simulink model "LKASampleSimulink"  (Simulink 9.1)
settings: Solver=ode1  StartTime=0.0  StopTime=inf  FixedStep=0.001  RelTol=1e-3
model workspace (MAT data in the model file):
  ParaDataStoreNum = Simulink.Parameter
  ParaDataStoreNum.DataType = 'int32'
  ParaDataStoreNum.Complexity = 'real'
  ParaDataStoreNum.Dimensions = [0 0]
InitFcn:
  | load('LKAExampleVariable.mat')
values from neighbouring files (symbols this model uses):
  DataStoreNumPara = 0    [LKAExampleVariable.mat]
  headwayOffset = 3.7    [LKAExampleVariable.mat]
undefined symbols (not defined in the file or in its folder): azimuth_angle, BrStatus, elevation_angle, GroundTruth_Objects, heading, id, Lane_Car_Distance_Left, Lane_Car_Distance_Right, Lane_Class, Lane_Coefficient_C0, Lane_Coefficient_C1, Lane_Coefficient_C2, Lane_Coefficient_C3, Lane_Curvature, Lane_Distance, Lane_ID, LaneInfoPerception, range_bbox, range_center, shape, time, Timestamp, type, velocity, width
libraries: mpcadaslib x1
(part 1 of 2)
Description:
  | 22222
settings Model: Creator=15751  LastModifiedBy=jwd  EnablePacing=on
settings DataIOCC: SaveFormat=Dataset  ReturnWorkspaceOutputs=on
settings DebuggingCC: UnderspecifiedInitializationDetection=Simplified  MergeDetectMultiDrivingBlocksExec=error  MultiTaskRateTransMsg=warning  SFUnexpectedBacktrackingDiag=error  SFNoUnconditionalDefaultTransitionDiag=error
settings HardwareCC: ProdBitPerPointer=64  ProdBitPerSizeT=64  ProdBitPerPtrDiffT=64  ProdLargestAtomicFloat=Float  ProdIntDivRoundTo=Zero  ProdEndianess=LittleEndian  ProdWordSize=64  ProdHWDeviceType=Intel->x86-64 (Windows64)
settings ModelReferenceCC: PropagateSignalLabelsOutOfModel=on
settings SFSimCC: SimUseLocalCustomCode=on
settings RTWCC: RTWUseLocalCustomCode=on
settings GRTTargetCC: TargetLangStandard=C99 (ISO)  CombineOutputUpdateFcns=on  GRTInterface=off
settings ConfigComp: CovMetricSettings=dwe  CovSaveCumulativeToWorkspaceVar=off  CovSaveSingleToWorkspaceVar=off  CovExternalEMLEnable=on

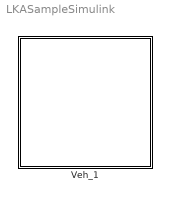
== system LKASampleSimulink ==
  Veh_1 : Subsystem  Tag=PanoSim_System
      mask Display: image(imread('Sedan_2.jpg'));color('white');text(0,0,'Veh_1','HorizontalAlignment','left','verticalAlignment','bottom');color('red');text(0.1,0.1,'P','HorizontalAlignment','right','verticalAlignment','top');

== system LKASampleSimulink/Veh_1 ==
  Algorithm : Subsystem
  AlgorithmControl : Subsystem
  ComplexVehicleModel : Subsystem
  Data Store Memory1 : DataStoreMemory  DataStoreName=DataStore_EGO_ALL  ReadBeforeWriteMsg=warning  WriteAfterWriteMsg=warning  WriteAfterReadMsg=warning  InitialValue=zeros(295,1)  ShowAdditionalParam=off  Dimensions=295
      settings: LockScale=on
  Data Store Memory2 : DataStoreMemory  DataStoreName=DataStore_COCKPIT_CONTROL  ReadBeforeWriteMsg=warning  WriteAfterWriteMsg=warning  WriteAfterReadMsg=warning  InitialValue=[0,0,0,0,0,0]  ShowAdditionalParam=off  Dimensions=6
      settings: LockScale=on
  Data Store Memory : DataStoreMemory  DataStoreName=DataStore_Ego_Control  ReadBeforeWriteMsg=warning  WriteAfterWriteMsg=warning  WriteAfterReadMsg=warning  InitialValue=[0,0,0,0,0,0]  ShowAdditionalParam=off  Dimensions=6
      settings: LockScale=on
  DriverModel : Subsystem  Tag=PanoSim_System
      mask Display: image(imread('driver.jpg'))
  GlobalVariable : Subsystem
  Sensors : Subsystem
  VehicleDataBus : Subsystem
  wires:
  Algorithm/3(LogDataOutput) -> VehicleDataBus/4(LogDataInput)
  Algorithm/2(GlobalVariableOutput) -> VehicleDataBus/2(GlobalVariable)
  Algorithm/1(ControlOutput) -> ComplexVehicleModel/1(Control)
  AlgorithmControl/1(AlgorithmControlOut) -> Algorithm/5(AlgorithmControlInput)
  GlobalVariable/1(Value) -> Algorithm/4(GlobalVariableInput)
  Sensors/1(SensorsOut) -> Algorithm/3(SensorsInput)
  DriverModel/1(DriverOut) -> Algorithm/2(ControlInput)
  [VehicleDynOut] -> Algorithm/1(VehDynInput)
  ComplexVehicleModel/1(Vehicle_Out) -> [VehicleDynOut], VehicleDataBus/1(VehicleDynOut)
  GlobalVariable/2(Original) -> VehicleDataBus/3(GlobalVariableOriginal)
  [VehicleDynOut] -> DriverModel/1(In1)

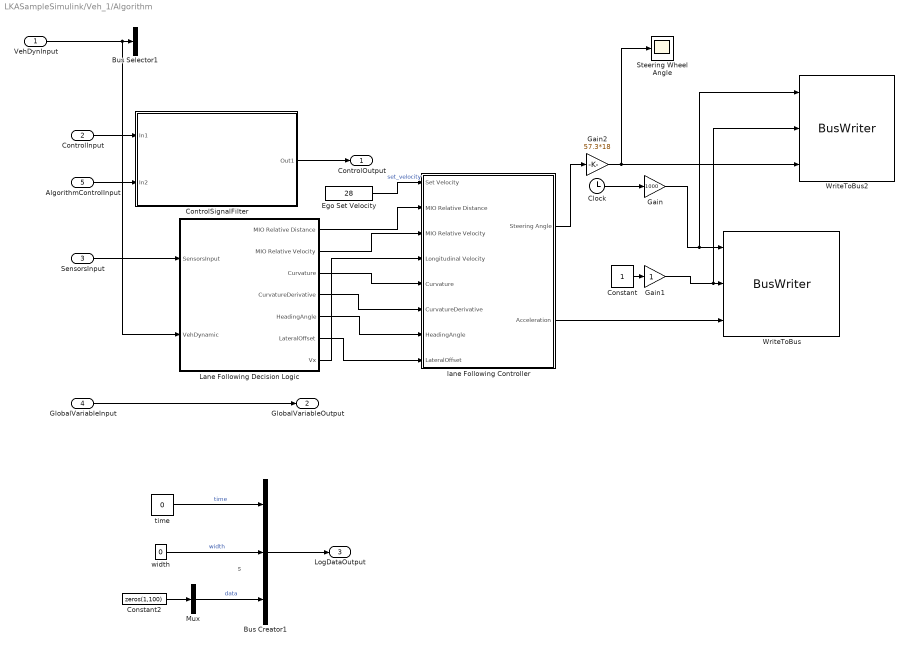
== system LKASampleSimulink/Veh_1/Algorithm ==
  note: s
  VehDynInput : Inport
  ControlInput : Inport  Port=2
  SensorsInput : Inport  Port=3
  GlobalVariableInput : Inport  Port=4
  AlgorithmControlInput : Inport  Port=5
  Bus Creator1 : BusCreator  Inputs=3
  Bus Selector1 : BusSelector  OutputSignals=ego
  Clock : Clock
  Constant : Constant
  Constant2 : Constant  Value=zeros(1,100)
  ControlSignalFilter : Subsystem
  Ego Set Velocity : Constant  Value=28  SampleTime=0.1
  Gain : Gain  Gain=1000  OutDataTypeStr=int32
  Gain1 : Gain  OutDataTypeStr=uint8
  Gain2 : Gain  Gain=57.3*18  OutDataTypeStr=double
  Lane Following Decision Logic : Subsystem
  Mux : Mux  Inputs=[100,]
  Steering Wheel Angle : Scope
  WriteToBus : S-Function  FunctionName=BusWriter  Parameters='xDriver_accel_input','time@i,valid@b,accel@d','0.01','0.0'  SFunctionDeploymentMode=off  EnableBusSupport=off
  WriteToBus2 : S-Function  FunctionName=BusWriter  Parameters='ego_control.steer','time@i,valid@b,steer@d','0.01','0.0'  SFunctionDeploymentMode=off  EnableBusSupport=off
  lane Following Controller : Subsystem
  time : Constant  Value=0
  width : Constant  Value=0
  ControlOutput : Outport  VectorParamsAs1DForOutWhenUnconnected=off
  GlobalVariableOutput : Outport  Port=2  VectorParamsAs1DForOutWhenUnconnected=off
  LogDataOutput : Outport  Port=3  VectorParamsAs1DForOutWhenUnconnected=off
  wires:
  VehDynInput/1 -> Lane Following Decision Logic/2(VehDynamic), Bus Selector1/1
  ControlInput/1 -> ControlSignalFilter/1(In1)
  ControlSignalFilter/1(Out1) -> ControlOutput/1
  GlobalVariableInput/1 -> GlobalVariableOutput/1
  time/1 -> Bus Creator1/1  "time"
  Bus Creator1/1 -> LogDataOutput/1
  Constant2/1 -> Mux/1
  Mux/1 -> Bus Creator1/3  "data"
  width/1 -> Bus Creator1/2  "width"
  AlgorithmControlInput/1 -> ControlSignalFilter/2(In2)
  Ego Set Velocity/1 -> lane Following Controller/1(Set Velocity)  "set_velocity"
  Lane Following Decision Logic/1(MIO Relative Distance) -> lane Following Controller/2(MIO Relative Distance)
  Lane Following Decision Logic/2(MIO Relative Velocity) -> lane Following Controller/3(MIO Relative Velocity)
  Lane Following Decision Logic/3(Curvature) -> lane Following Controller/5(Curvature)
  Lane Following Decision Logic/6(LateralOffset) -> lane Following Controller/8(LateralOffset)
  SensorsInput/1 -> Lane Following Decision Logic/1(SensorsInput)
  lane Following Controller/1(Steering Angle) -> Gain2/1
  lane Following Controller/2(Acceleration) -> WriteToBus/3
  Gain/1 -> WriteToBus2/1, WriteToBus/1
  Clock/1 -> Gain/1
  Gain1/1 -> WriteToBus2/2, WriteToBus/2
  Constant/1 -> Gain1/1
  Lane Following Decision Logic/7(Vx) -> lane Following Controller/4(Longitudinal Velocity)
  Lane Following Decision Logic/5(HeadingAngle) -> lane Following Controller/7(HeadingAngle)
  Lane Following Decision Logic/4(CurvatureDerivative) -> lane Following Controller/6(CurvatureDerivative)
  Gain2/1 -> Steering Wheel Angle/1, WriteToBus2/3

== system LKASampleSimulink/Veh_1/AlgorithmControl ==
  Bus{,2..5} (5 alike) : BusCreator  Inputs=3
  Bus1 : BusCreator  Inputs=5
  brake : S-Function  FunctionName=BusReader  Parameters='ego_control.brake','time@i,valid@b,brake@d','0.001','0.0'  SFunctionDeploymentMode=off  EnableBusSupport=off
  gear : S-Function  FunctionName=BusReader  Parameters='ego_control.gear','time@i,valid@b,gear@i','0.001','0.0'  SFunctionDeploymentMode=off  EnableBusSupport=off
  mode : S-Function  FunctionName=BusReader  Parameters='ego_control.mode','time@i,valid@b,mode@i','0.001','0.0'  SFunctionDeploymentMode=off  EnableBusSupport=off
  steer : S-Function  FunctionName=BusReader  Parameters='ego_control.steer','time@i,valid@b,steer@d','0.001','0.0'  SFunctionDeploymentMode=off  EnableBusSupport=off
  throttle : S-Function  FunctionName=BusReader  Parameters='ego_control.throttle','time@i,valid@b,throttle@d','0.001','0.0'  SFunctionDeploymentMode=off  EnableBusSupport=off
  AlgorithmControlOut : Outport  VectorParamsAs1DForOutWhenUnconnected=off
  wires:
  Bus1/1 -> AlgorithmControlOut/1
  Bus5/1 -> Bus1/1  "throttle"
  Bus4/1 -> Bus1/5  "gear"
  Bus3/1 -> Bus1/4  "mode"
  Bus2/1 -> Bus1/3  "steer"
  Bus/1 -> Bus1/2  "brake"
  gear/3 -> Bus4/3  "value"
  gear/2 -> Bus4/2  "valid"
  gear/1 -> Bus4/1  "time"
  mode/3 -> Bus3/3  "value"
  mode/2 -> Bus3/2  "valid"
  mode/1 -> Bus3/1  "time"
  steer/1 -> Bus2/1  "time"
  brake/1 -> Bus/1  "time"
  throttle/1 -> Bus5/1  "time"
  throttle/3 -> Bus5/3  "value"
  brake/3 -> Bus/3  "value"
  steer/3 -> Bus2/3  "value"
  throttle/2 -> Bus5/2  "valid"
  brake/2 -> Bus/2  "valid"
  steer/2 -> Bus2/2  "valid"

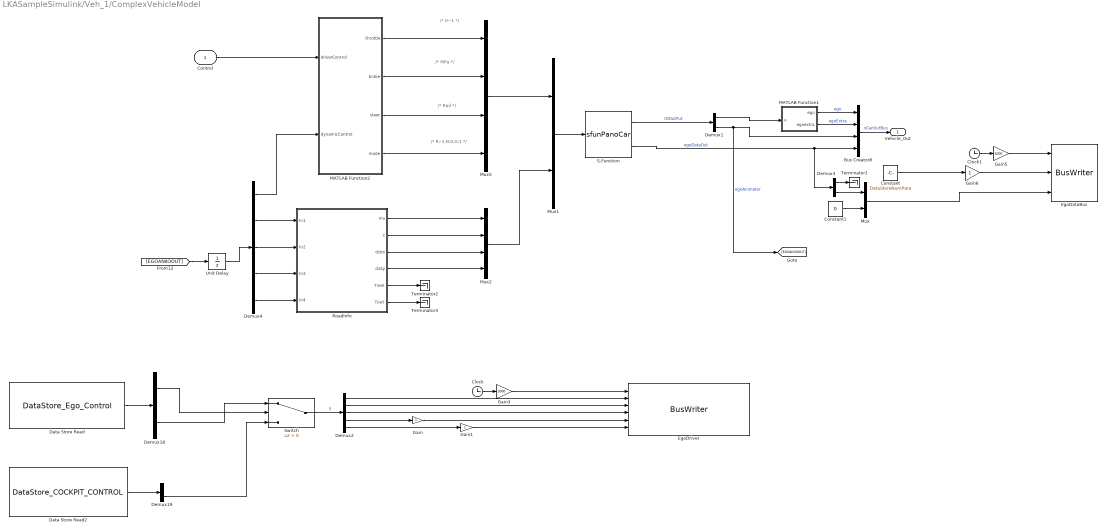
== system LKASampleSimulink/Veh_1/ComplexVehicleModel ==
  note: /* MPa */
  note: /* 0~1 */
  note: /* R:-1,N:0,D:1 */
  note: /* Rad */
  Control : Inport
  Bus Creator8 : BusCreator  Inputs=4
  Clock : Clock
  Clock1 : Clock
  Constant : Constant  Value=DataStoreNumPara  VectorParams1D=off  OutDataTypeStr=double
  Constant1 : Constant  Value=0
  Data Store Read : DataStoreRead  DataStoreName=DataStore_Ego_Control
  Data Store Read2 : DataStoreRead  DataStoreName=DataStore_COCKPIT_CONTROL
  Demux1 : Demux  Outputs=[19,57]
  Demux18 : Demux  Outputs=[1,5]
  Demux19 : Demux  Outputs=[1,5]
  Demux2 : Demux  Outputs=5
  Demux3 : Demux  Outputs=[1,499]
  Demux4 : Demux  Outputs=[5,13,13,13,13]
  EgoDataBus : S-Function  FunctionName=BusWriter  Parameters='ego_data','time@i,500@[,data@d','0.01','0.0'  SFunctionDeploymentMode=off  EnableBusSupport=off
  EgoDriver : S-Function  FunctionName=BusWriter  Parameters='ego_driver','time@i,throttle@d,brake@d,steer@d,mode@i,gear@i','0.01','0.0'  SFunctionDeploymentMode=off  EnableBusSupport=off
  Gain : Gain  OutDataTypeStr=int32
  Gain1 : Gain  OutDataTypeStr=int32
  Gain3 : Gain  Gain=1000  OutDataTypeStr=Inherit: Inherit via back propagation  RndMeth=Nearest
  Gain5 : Gain  Gain=1000  OutDataTypeStr=Inherit: Inherit via back propagation  RndMeth=Nearest
  Gain6 : Gain  OutDataTypeStr=int32
  MATLAB Function1 : MATLAB Function  TreatAsAtomicUnit=on
  MATLAB Function2 : MATLAB Function  TreatAsAtomicUnit=on
  Mux : Mux  Inputs=[499,1]
  Mux1 : Mux  Inputs=[4,16]
  Mux2 : Mux
  Mux5 : Mux
  RoadInfo : Subsystem
  S-Function : S-Function  FunctionName=sfunPanoCar  SFunctionDeploymentMode=off  EnableBusSupport=off
  Switch : Switch  Criteria=u2 > Threshold
  Terminator1 : Terminator
  Terminator2 : Terminator
  Terminator3 : Terminator
  Unit Delay : UnitDelay  SampleTime=-1  HasFrameUpgradeWarning=on
  Vehicle_Out : Outport
  wires:
  Demux19/2 -> Switch/3
  Demux18/2 -> Switch/1
  Demux18/1 -> Switch/2
  MATLAB Function2/4(mode) -> Mux5/4
  MATLAB Function2/3(steer) -> Mux5/3
  MATLAB Function2/2(brake) -> Mux5/2
  MATLAB Function2/1(throttle) -> Mux5/1
  Demux4/4 -> RoadInfo/3(In3)
  Demux4/1 -> MATLAB Function2/2(dynamicControl)
  Demux4/2 -> RoadInfo/1(In1)
  Demux4/5 -> RoadInfo/4(In4)
  Unit Delay/1 -> Demux4/1
  Demux4/3 -> RoadInfo/2(In2)
  Mux/1 -> EgoDataBus/3
  Constant1/1 -> Mux/2
  Demux3/2 -> Mux/1
  Demux3/1 -> Terminator1/1
  Constant/1 -> Gain6/1
  Gain5/1 -> EgoDataBus/1
  Clock1/1 -> Gain5/1
  Gain6/1 -> EgoDataBus/2
  Data Store Read2/1 -> Demux19/1
  Data Store Read/1 -> Demux18/1
  Switch/1 -> Demux2/1  "5"
  Demux1/2 -> Bus Creator8/3, [EGOANIIOOUT]  "egoAnimator"
  MATLAB Function1/1(ego) -> Bus Creator8/1  "ego"
  Demux1/1 -> MATLAB Function1/1(u)
  MATLAB Function1/2(egoextra) -> Bus Creator8/2  "egoExtra"
  RoadInfo/6(TireY) -> Terminator3/1
  RoadInfo/5(TireX) -> Terminator2/1
  S-Function/2 -> Bus Creator8/4, Demux3/1  "egoDataOut"
  Gain1/1 -> EgoDriver/6
  Gain/1 -> EgoDriver/5
  Demux2/4 -> Gain/1
  Demux2/2 -> EgoDriver/3
  Control/1 -> MATLAB Function2/1(driverControl)
  Demux2/1 -> EgoDriver/2
  Demux2/3 -> EgoDriver/4
  Demux2/5 -> Gain1/1
  Gain3/1 -> EgoDriver/1
  Mux1/1 -> S-Function/1
  S-Function/1 -> Demux1/1  "IOOutPut"
  Bus Creator8/1 -> Vehicle_Out/1  "xCarOutBus"
  Mux5/1 -> Mux1/1
  Clock/1 -> Gain3/1
  Mux2/1 -> Mux1/2
  RoadInfo/3(dzdx) -> Mux2/3
  RoadInfo/1(mu) -> Mux2/1
  RoadInfo/2(z) -> Mux2/2
  RoadInfo/4(dzdy) -> Mux2/4
  [EGOANIIOOUT] -> Unit Delay/1

== system LKASampleSimulink/Veh_1/DriverModel ==
  In1 : Inport
  DriverFilter : Subsystem
  DriverOut : Outport  VectorParamsAs1DForOutWhenUnconnected=off
  wires:
  DriverFilter/1(DriverOut) -> DriverOut/1

== system LKASampleSimulink/Veh_1/GlobalVariable ==
  Bus : BusCreator  Inputs=2
  Variable : Subsystem
  Value : Outport  VectorParamsAs1DForOutWhenUnconnected=off
  Original : Outport  Port=2  VectorParamsAs1DForOutWhenUnconnected=off
  wires:
  Bus/1 -> Original/1
  Variable/2(Out2) -> Bus/2  "Time"
  Variable/1(Out1) -> Value/1, Bus/1  "Value"

== system LKASampleSimulink/Veh_1/Sensors ==
  GroundTruth_Objects.0 : Subsystem
  LaneInfoPerception.0 : Subsystem
  SensorsBusCreator : BusCreator  Inputs=LaneInfoPerception.0,GroundTruth_Objects.0
  sensor_template : Subsystem  Commented=on
  SensorsOut : Outport  VectorParamsAs1DForOutWhenUnconnected=off
  wires:
  SensorsBusCreator/1 -> SensorsOut/1
  GroundTruth_Objects.0/1(SensorOut) -> SensorsBusCreator/2  "GroundTruth_Objects.0"
  LaneInfoPerception.0/1(SensorOut) -> SensorsBusCreator/1  "LaneInfoPerception.0"

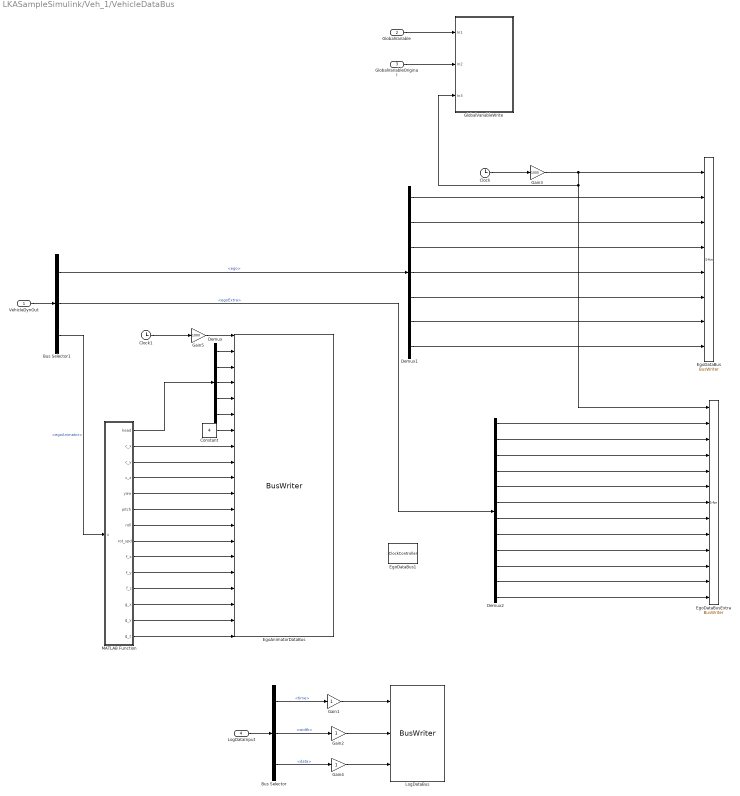
== system LKASampleSimulink/Veh_1/VehicleDataBus ==
  VehicleDynOut : Inport
  GlobalVariable : Inport  Port=2
  GlobalVariableOriginal : Inport  Port=3
  LogDataInput : Inport  Port=4
  Bus Selector : BusSelector  OutputSignals=time,width,data
  Bus Selector1 : BusSelector  OutputSignals=ego,egoExtra,egoAnimator
  Clock : Clock
  Clock1 : Clock
  Constant : Constant  Value=4  OutDataTypeStr=int32
  Demux : Demux  Outputs=5
  Demux1 : Demux  Outputs=7
  Demux2 : Demux  Outputs=12
  EgoAnimatorDataBus : S-Function  FunctionName=BusWriter  Parameters='ego_animator','time@i,rot_spd@d,trans_gear@d,throttle@d,master@d,str@d,4@[,center_x@d,center_y@d,center_z@d,yaw@d,pitch@d,roll@d,rotation_spd@d,force_tire_x@d,force_tire_y@d,force_tire_z@d,gnd_x@d,gnd_y@d,gnd_z@d','0.01','0.0'  SFunctionDeploymentMode=off  EnableBusSupport=off
  EgoDataBus : S-Function  FunctionName=BusWriter  Parameters='ego','time@i,x@d,y@d,z@d,yaw@d,pitch@d,roll@d,speed@d','0.01','0.0'  SFunctionDeploymentMode=off  EnableBusSupport=off
  EgoDataBus1 : S-Function  FunctionName=ClockController  Parameters='step','0.01','0.0'  SFunctionDeploymentMode=off  EnableBusSupport=off
  EgoDataBusExtra : S-Function  FunctionName=BusWriter  Parameters='ego_extra','time@i,VX@d,VY@d,VZ@d,AVx@d,AVy@d,AVz@d,Ax@d,Ay@d,Az@d,AAx@d,AAy@d,AAz@d','0.01','0.0'  SFunctionDeploymentMode=off  EnableBusSupport=off
  Gain1 : Gain  OutDataTypeStr=int32  RndMeth=Nearest
  Gain2 : Gain  OutDataTypeStr=int32  RndMeth=Nearest
  Gain3 : Gain  Gain=1000  OutDataTypeStr=Inherit: Inherit via back propagation  RndMeth=Nearest
  Gain4 : Gain  OutDataTypeStr=double  RndMeth=Nearest
  Gain5 : Gain  Gain=1000  OutDataTypeStr=Inherit: Inherit via back propagation  RndMeth=Nearest
  GlobalVariableWrite : Subsystem
  LogDataBus : S-Function  FunctionName=BusWriter  Parameters='data','time@i,100@[,data@d','0.01','0.0'  SFunctionDeploymentMode=off  EnableBusSupport=off
  MATLAB Function : MATLAB Function  TreatAsAtomicUnit=on
  wires:
  Demux/5 -> EgoAnimatorDataBus/6
  MATLAB Function/14(g_z) -> EgoAnimatorDataBus/20
  MATLAB Function/13(g_y) -> EgoAnimatorDataBus/19
  MATLAB Function/12(g_x) -> EgoAnimatorDataBus/18
  MATLAB Function/11(f_z) -> EgoAnimatorDataBus/17
  MATLAB Function/10(f_y) -> EgoAnimatorDataBus/16
  MATLAB Function/9(f_x) -> EgoAnimatorDataBus/15
  MATLAB Function/8(rot_spd) -> EgoAnimatorDataBus/14
  MATLAB Function/7(roll) -> EgoAnimatorDataBus/13
  MATLAB Function/6(pitch) -> EgoAnimatorDataBus/12
  MATLAB Function/5(yaw) -> EgoAnimatorDataBus/11
  MATLAB Function/4(c_z) -> EgoAnimatorDataBus/10
  MATLAB Function/3(c_y) -> EgoAnimatorDataBus/9
  MATLAB Function/2(c_x) -> EgoAnimatorDataBus/8
  Constant/1 -> EgoAnimatorDataBus/7
  Demux/4 -> EgoAnimatorDataBus/5
  Demux/3 -> EgoAnimatorDataBus/4
  Demux/2 -> EgoAnimatorDataBus/3
  Demux/1 -> EgoAnimatorDataBus/2
  MATLAB Function/1(head) -> Demux/1
  Gain5/1 -> EgoAnimatorDataBus/1
  Clock1/1 -> Gain5/1
  Bus Selector1/3 -> MATLAB Function/1(u)  "<egoAnimator>"
  Bus Selector1/2 -> Demux2/1  "<egoExtra>"
  Bus Selector1/1 -> Demux1/1  "<ego>"
  Gain2/1 -> LogDataBus/2
  Bus Selector/2 -> Gain2/1  "<width>"
  Gain4/1 -> LogDataBus/3
  Bus Selector/1 -> Gain1/1  "<time>"
  Bus Selector/3 -> Gain4/1  "<data>"
  Gain1/1 -> LogDataBus/1
  LogDataInput/1 -> Bus Selector/1
  GlobalVariableOriginal/1 -> GlobalVariableWrite/2(In2)
  Gain3/1 -> EgoDataBus/1, EgoDataBusExtra/1, GlobalVariableWrite/3(In3)
  GlobalVariable/1 -> GlobalVariableWrite/1(In1)
  Demux2/12 -> EgoDataBusExtra/13
  Demux2/11 -> EgoDataBusExtra/12
  Demux2/10 -> EgoDataBusExtra/11
  Demux2/9 -> EgoDataBusExtra/10
  Demux2/8 -> EgoDataBusExtra/9
  Demux2/7 -> EgoDataBusExtra/8
  Demux2/6 -> EgoDataBusExtra/7
  Demux2/5 -> EgoDataBusExtra/6
  Demux2/4 -> EgoDataBusExtra/5
  Demux2/3 -> EgoDataBusExtra/4
  Demux2/2 -> EgoDataBusExtra/3
  Demux2/1 -> EgoDataBusExtra/2
  VehicleDynOut/1 -> Bus Selector1/1
  Clock/1 -> Gain3/1
  Demux1/1 -> EgoDataBus/2
  Demux1/2 -> EgoDataBus/3
  Demux1/3 -> EgoDataBus/4
  Demux1/4 -> EgoDataBus/5
  Demux1/5 -> EgoDataBus/6
  Demux1/6 -> EgoDataBus/7
  Demux1/7 -> EgoDataBus/8

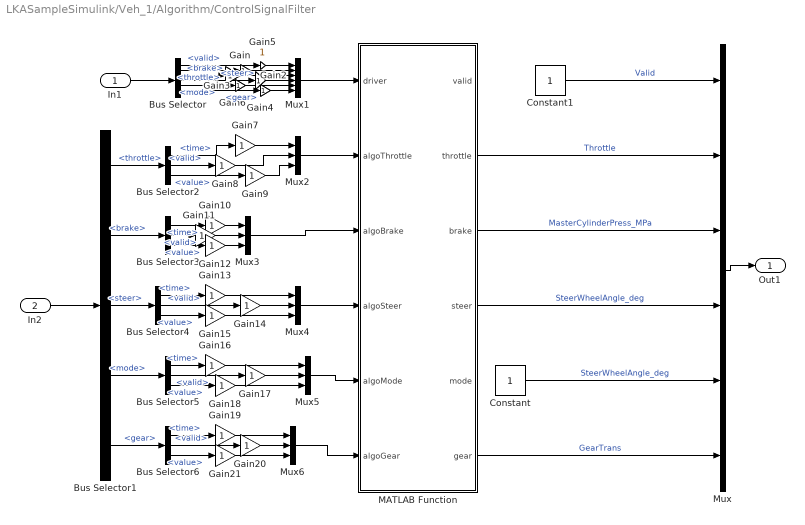
== system LKASampleSimulink/Veh_1/Algorithm/ControlSignalFilter ==
  In1 : Inport
  In2 : Inport  Port=2
  Bus Selector : BusSelector  OutputSignals=valid,throttle,brake,steer,mode,gear
  Bus Selector1 : BusSelector  OutputSignals=throttle,brake,steer,mode,gear
  Bus Selector{2..6} (5 alike) : BusSelector  OutputSignals=time,valid,value
  Constant : Constant
  Constant1 : Constant
  Gain{,2..21} (21 alike) : Gain  OutDataTypeStr=double
  MATLAB Function : MATLAB Function  TreatAsAtomicUnit=on
  Mux : Mux  Inputs=6
  Mux1 : Mux  Inputs=6
  Mux{2..6} (5 alike) : Mux  Inputs=3
  Out1 : Outport  VectorParamsAs1DForOutWhenUnconnected=off
  wires:
  In1/1 -> Bus Selector/1
  Mux/1 -> Out1/1
  MATLAB Function/2(throttle) -> Mux/2  "Throttle"
  MATLAB Function/4(steer) -> Mux/4  "SteerWheelAngle_deg"
  Constant1/1 -> Mux/1  "Valid"
  MATLAB Function/6(gear) -> Mux/6  "GearTrans"
  In2/1 -> Bus Selector1/1
  Bus Selector1/1 -> Bus Selector2/1  "<throttle>"
  Bus Selector1/2 -> Bus Selector3/1  "<brake>"
  Bus Selector1/3 -> Bus Selector4/1  "<steer>"
  Bus Selector1/4 -> Bus Selector5/1  "<mode>"
  Bus Selector1/5 -> Bus Selector6/1  "<gear>"
  MATLAB Function/3(brake) -> Mux/3  "MasterCylinderPress_MPa"
  Bus Selector/1 -> Gain5/1  "<valid>"
  Bus Selector/2 -> Gain/1  "<throttle>"
  Bus Selector/3 -> Gain6/1  "<brake>"
  Bus Selector/4 -> Gain4/1  "<steer>"
  Bus Selector/5 -> Gain3/1  "<mode>"
  Bus Selector/6 -> Gain2/1  "<gear>"
  Mux1/1 -> MATLAB Function/1(driver)
  Bus Selector2/1 -> Gain7/1  "<time>"
  Bus Selector2/2 -> Gain8/1  "<valid>"
  Bus Selector2/3 -> Gain9/1  "<value>"
  Mux2/1 -> MATLAB Function/2(algoThrottle)
  Bus Selector3/1 -> Gain10/1  "<time>"
  Bus Selector3/2 -> Gain11/1  "<valid>"
  Bus Selector3/3 -> Gain12/1  "<value>"
  Mux3/1 -> MATLAB Function/3(algoBrake)
  Bus Selector4/1 -> Gain13/1  "<time>"
  Bus Selector4/2 -> Gain14/1  "<valid>"
  Bus Selector4/3 -> Gain15/1  "<value>"
  Mux4/1 -> MATLAB Function/4(algoSteer)
  Bus Selector5/1 -> Gain16/1  "<time>"
  Bus Selector5/2 -> Gain17/1  "<valid>"
  Bus Selector5/3 -> Gain18/1  "<value>"
  Mux5/1 -> MATLAB Function/5(algoMode)
  Bus Selector6/1 -> Gain19/1  "<time>"
  Bus Selector6/2 -> Gain20/1  "<valid>"
  Bus Selector6/3 -> Gain21/1  "<value>"
  Mux6/1 -> MATLAB Function/6(algoGear)
  Gain/1 -> Mux1/2
  Gain2/1 -> Mux1/6
  Gain3/1 -> Mux1/5
  Gain4/1 -> Mux1/4
  Gain5/1 -> Mux1/1
  Gain6/1 -> Mux1/3
  Gain7/1 -> Mux2/1
  Gain8/1 -> Mux2/2
  Gain9/1 -> Mux2/3
  Gain10/1 -> Mux3/1
  Gain11/1 -> Mux3/2
  Gain12/1 -> Mux3/3
  Gain13/1 -> Mux4/1
  Gain14/1 -> Mux4/2
  Gain15/1 -> Mux4/3
  Gain16/1 -> Mux5/1
  Gain17/1 -> Mux5/2
  Gain18/1 -> Mux5/3
  Gain19/1 -> Mux6/1
  Gain20/1 -> Mux6/2
  Gain21/1 -> Mux6/3
  Constant/1 -> Mux/5  "SteerWheelAngle_deg"

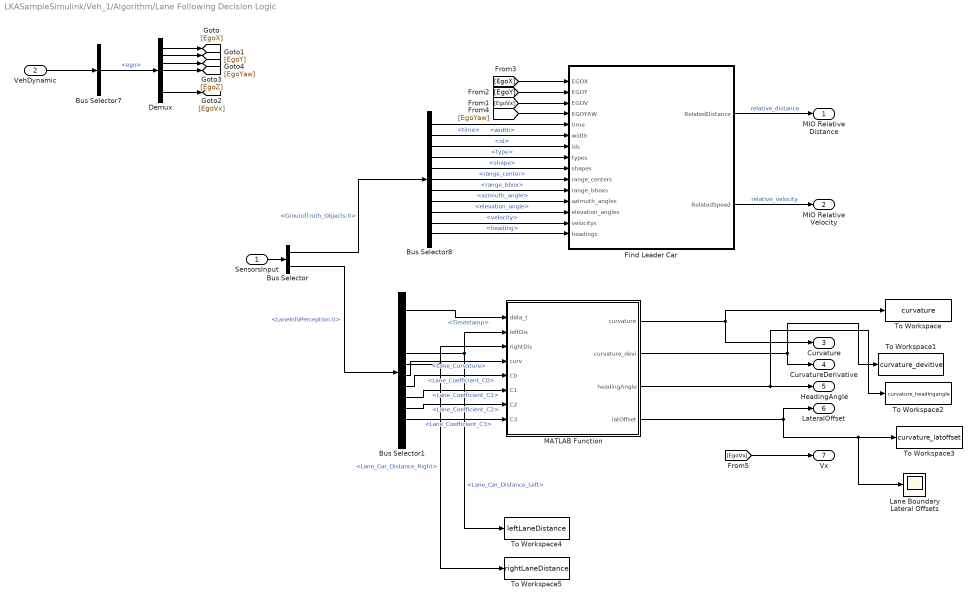
== system LKASampleSimulink/Veh_1/Algorithm/Lane Following Decision Logic ==
  SensorsInput : Inport
  VehDynamic : Inport  Port=2
  Bus Selector : BusSelector  OutputSignals=GroundTruth_Objects:0,LaneInfoPerception:0
  Bus Selector1 : BusSelector  OutputSignals=Timestamp,width,Lane_ID,Lane_Distance,Lane_Car_Distance_Left,Lane_Car_Distance_Right,Lane_Curvature,Lane_Coefficient_C0,Lane_Coefficient_C1,Lane_Coefficient_C2,Lane_Coefficient_C3,Lane_Class
  Bus Selector7 : BusSelector  OutputSignals=ego
  Bus Selector8 : BusSelector  OutputSignals=time,width,id,type,shape,range_center,range_bbox,azimuth_angle,elevation_angle,velocity,heading
  Demux : Demux  Outputs=[1,1,1,1,1,1,1]
  Find Leader Car : MATLAB Function  TreatAsAtomicUnit=on
  Lane Boundary Lateral Offsets : Scope
  MATLAB Function : MATLAB Function  TreatAsAtomicUnit=on
  To Workspace : ToWorkspace  VariableName=curvature  SaveFormat=Timeseries  SampleTime=-1
  To Workspace1 : ToWorkspace  VariableName=curvature_devitive  SaveFormat=Timeseries  SampleTime=-1
  To Workspace2 : ToWorkspace  VariableName=curvature_headingangle  SaveFormat=Timeseries  SampleTime=-1
  To Workspace3 : ToWorkspace  VariableName=curvature_latoffset  SaveFormat=Timeseries  SampleTime=-1
  To Workspace4 : ToWorkspace  VariableName=leftLaneDistance  SaveFormat=Timeseries  SampleTime=-1
  To Workspace5 : ToWorkspace  VariableName=rightLaneDistance  SaveFormat=Timeseries  SampleTime=-1
  MIO Relative Distance : Outport
  MIO Relative Velocity : Outport  Port=2
  Curvature : Outport  Port=3  OutDataTypeStr=double
  CurvatureDerivative : Outport  Port=4  OutDataTypeStr=double
  HeadingAngle : Outport  Port=5  OutDataTypeStr=double
  LateralOffset : Outport  Port=6  OutDataTypeStr=double
  Vx : Outport  Port=7  OutDataTypeStr=double
  wires:
  Find Leader Car/1(RelatedDistance) -> MIO Relative Distance/1  "relative_distance"
  Find Leader Car/2(RelatedSpeed) -> MIO Relative Velocity/1  "relative_velocity"
  SensorsInput/1 -> Bus Selector/1
  Demux/4 -> [EgoYaw]
  VehDynamic/1 -> Bus Selector7/1
  Demux/7 -> [EgoVx]
  Demux/1 -> [EgoX]
  Demux/3 -> [EgoZ]
  Bus Selector7/1 -> Demux/1  "<ego>"
  Demux/2 -> [EgoY]
  Bus Selector8/6 -> Find Leader Car/10(range_centers)  "<range_center>"
  Bus Selector8/2 -> Find Leader Car/6(width)  "<width>"
  Bus Selector8/10 -> Find Leader Car/14(velocitys)  "<velocity>"
  Bus Selector8/8 -> Find Leader Car/12(azimuth_angles)  "<azimuth_angle>"
  Bus Selector8/9 -> Find Leader Car/13(elevation_angles)  "<elevation_angle>"
  Bus Selector8/1 -> Find Leader Car/5(time)  "<time>"
  Bus Selector8/3 -> Find Leader Car/7(ids)  "<id>"
  [EgoYaw] -> Find Leader Car/4(EGOYAW)
  Bus Selector8/4 -> Find Leader Car/8(types)  "<type>"
  Bus Selector8/5 -> Find Leader Car/9(shapes)  "<shape>"
  Bus Selector8/7 -> Find Leader Car/11(range_bboxs)  "<range_bbox>"
  Bus Selector8/11 -> Find Leader Car/15(headings)  "<heading>"
  [EgoX] -> Find Leader Car/1(EGOX)
  [EgoVx] -> Find Leader Car/3(EGOV)
  [EgoY] -> Find Leader Car/2(EGOY)
  Bus Selector/1 -> Bus Selector8/1  "<GroundTruth_Objects:0>"
  Bus Selector/2 -> Bus Selector1/1  "<LaneInfoPerception:0>"
  Bus Selector1/6 -> To Workspace5/1, MATLAB Function/3(rightDis)  "<Lane_Car_Distance_Right>"
  MATLAB Function/1(curvature) -> To Workspace/1, Curvature/1
  MATLAB Function/2(curvature_devi) -> To Workspace1/1, CurvatureDerivative/1
  MATLAB Function/3(headingAngle) -> To Workspace2/1, HeadingAngle/1
  MATLAB Function/4(latOffset) -> LateralOffset/1, Lane Boundary Lateral Offsets/1, To Workspace3/1
  Bus Selector1/5 -> To Workspace4/1, MATLAB Function/2(leftDis)  "<Lane_Car_Distance_Left>"
  Bus Selector1/7 -> MATLAB Function/4(curv)  "<Lane_Curvature>"
  Bus Selector1/8 -> MATLAB Function/5(C0)  "<Lane_Coefficient_C0>"
  Bus Selector1/9 -> MATLAB Function/6(C1)  "<Lane_Coefficient_C1>"
  Bus Selector1/10 -> MATLAB Function/7(C2)  "<Lane_Coefficient_C2>"
  Bus Selector1/11 -> MATLAB Function/8(C3)  "<Lane_Coefficient_C3>"
  [EgoVx] -> Vx/1
  Bus Selector1/1 -> MATLAB Function/1(data_t)  "<Timestamp>"

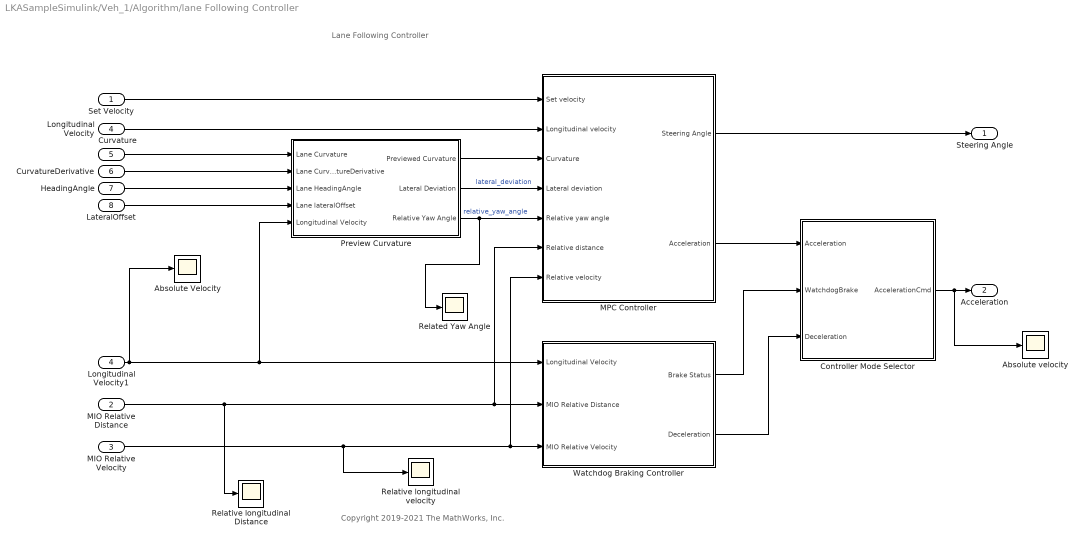
== system LKASampleSimulink/Veh_1/Algorithm/lane Following Controller ==
  note: Copyright 2019-2021 The MathWorks, Inc.
  note: Lane Following Controller
  Set Velocity : Inport
  MIO Relative Distance : Inport  Port=2
  MIO Relative Velocity : Inport  Port=3
  Longitudinal Velocity : Inport  Port=4
  Curvature : Inport  Port=5  OutDataTypeStr=double
  CurvatureDerivative : Inport  Port=6  OutDataTypeStr=double
  HeadingAngle : Inport  Port=7  OutDataTypeStr=double
  LateralOffset : Inport  Port=8  OutDataTypeStr=double
  Absolute Velocity : Scope
  Absolute velocity : Scope
  Controller Mode Selector : Subsystem
  Longitudinal Velocity1 : InportShadow  Port=4
  MPC Controller : Subsystem
  Preview Curvature : Subsystem  VariantControl=v2
      settings: RTWFileNameOpts=Use function name
  Related Yaw Angle : Scope
  Relative longitudinal Distance : Scope
  Relative longitudinal velocity : Scope
  Watchdog Braking Controller : Subsystem
  Steering Angle : Outport  PortDimensions=1  VectorParamsAs1DForOutWhenUnconnected=off
  Acceleration : Outport  Port=2  PortDimensions=1  VectorParamsAs1DForOutWhenUnconnected=off
  wires:
  Preview Curvature/2(Lateral Deviation) -> MPC Controller/4(Lateral deviation)  "lateral_deviation"
  Curvature/1 -> Preview Curvature/1(Lane Curvature)
  MPC Controller/2(Acceleration) -> Controller Mode Selector/1(Acceleration)
  MIO Relative Distance/1 -> Relative longitudinal Distance/1, Watchdog Braking Controller/2(MIO Relative Distance), MPC Controller/6(Relative distance)
  Preview Curvature/1(Previewed Curvature) -> MPC Controller/3(Curvature)
  MIO Relative Velocity/1 -> Relative longitudinal velocity/1, MPC Controller/7(Relative velocity), Watchdog Braking Controller/3(MIO Relative Velocity)
  Longitudinal Velocity/1 -> MPC Controller/2(Longitudinal velocity)
  Set Velocity/1 -> MPC Controller/1(Set velocity)
  Watchdog Braking Controller/1(Brake Status) -> Controller Mode Selector/2(WatchdogBrake)
  Preview Curvature/3(Relative Yaw Angle) -> Related Yaw Angle/1, MPC Controller/5(Relative yaw angle)  "relative_yaw_angle"
  MPC Controller/1(Steering Angle) -> Steering Angle/1
  Watchdog Braking Controller/2(Deceleration) -> Controller Mode Selector/3(Deceleration)
  Controller Mode Selector/1(AccelerationCmd) -> Absolute velocity/1, Acceleration/1
  CurvatureDerivative/1 -> Preview Curvature/2(Lane CurvatureDerivative)
  HeadingAngle/1 -> Preview Curvature/3(Lane HeadingAngle)
  LateralOffset/1 -> Preview Curvature/4(Lane lateralOffset)
  Longitudinal Velocity1/1 -> Preview Curvature/5(Longitudinal Velocity), Watchdog Braking Controller/1(Longitudinal Velocity), Absolute Velocity/1

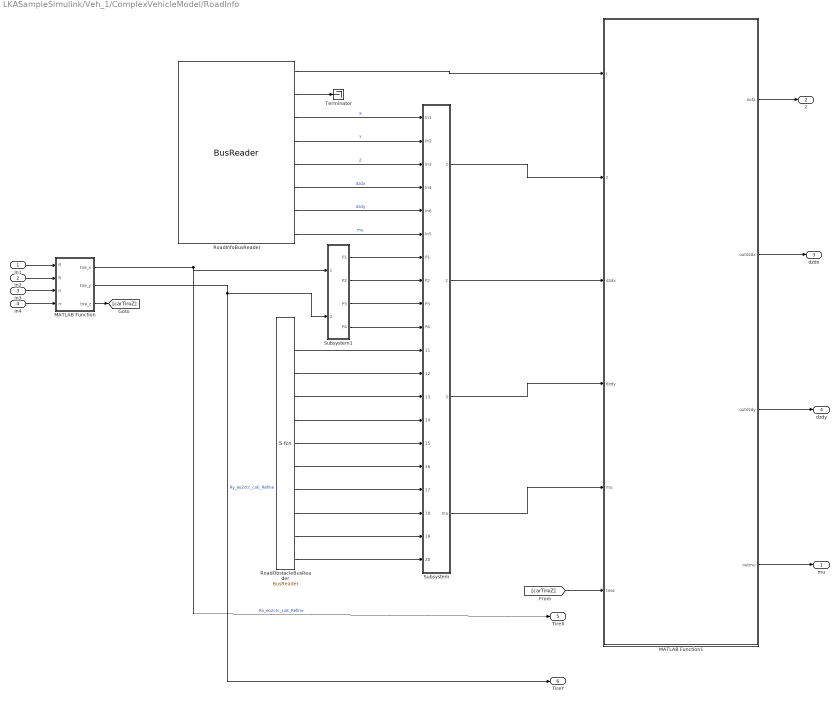
== system LKASampleSimulink/Veh_1/ComplexVehicleModel/RoadInfo ==
  In1 : Inport
  In2 : Inport  Port=2
  In3 : Inport  Port=3
  In4 : Inport  Port=4
  MATLAB Function : MATLAB Function  TreatAsAtomicUnit=on
  MATLAB Function1 : MATLAB Function  TreatAsAtomicUnit=on
  RoadInfoBusReader : S-Function  FunctionName=BusReader  Parameters='road_info','time@i,16@[,x@d,y@d,z@d,dzdx@d,dzdy@d,mu@d','0.001','0.0'  SFunctionDeploymentMode=off  EnableBusSupport=off
  RoadObstacleBusReader : S-Function  FunctionName=BusReader  Parameters='road_obstacle','time@i,4@[,x1@d,y1@d,x2@d,y2@d,x3@d,y3@d,x4@d,y4@d,z@d','0.001','0.0'  SFunctionDeploymentMode=off  EnableBusSupport=off
  Subsystem : Subsystem
  Subsystem1 : Subsystem
  Terminator : Terminator
  mu : Outport  VectorParamsAs1DForOutWhenUnconnected=off
  z : Outport  Port=2  VectorParamsAs1DForOutWhenUnconnected=off
  dzdx : Outport  Port=3  VectorParamsAs1DForOutWhenUnconnected=off
  dzdy : Outport  Port=4  VectorParamsAs1DForOutWhenUnconnected=off
  TireX : Outport  Port=5  VectorParamsAs1DForOutWhenUnconnected=off
  TireY : Outport  Port=6  VectorParamsAs1DForOutWhenUnconnected=off
  wires:
  In1/1 -> MATLAB Function/1(fl)
  In2/1 -> MATLAB Function/2(fr)
  In3/1 -> MATLAB Function/3(rl)
  In4/1 -> MATLAB Function/4(rr)
  MATLAB Function1/4(outmu) -> mu/1
  MATLAB Function1/3(outdzdy) -> dzdy/1
  MATLAB Function1/2(outdzdx) -> dzdx/1
  MATLAB Function1/1(outz) -> z/1
  [carTireZ] -> MATLAB Function1/6(tirez)
  RoadInfoBusReader/1 -> MATLAB Function1/1(t)
  RoadInfoBusReader/2 -> Terminator/1
  MATLAB Function/3(tire_z) -> [carTireZ]
  RoadObstacleBusReader/11 -> Subsystem/20(In20)
  RoadObstacleBusReader/10 -> Subsystem/19(In19)
  RoadObstacleBusReader/9 -> Subsystem/18(In18)
  RoadObstacleBusReader/8 -> Subsystem/17(In17)
  RoadObstacleBusReader/7 -> Subsystem/16(In16)
  RoadObstacleBusReader/6 -> Subsystem/15(In15)
  RoadObstacleBusReader/5 -> Subsystem/14(In14)
  RoadObstacleBusReader/4 -> Subsystem/13(In13)
  RoadObstacleBusReader/3 -> Subsystem/12(In12)
  RoadObstacleBusReader/2 -> Subsystem/11(In11)
  RoadInfoBusReader/3 -> Subsystem/1(In1)  "X"
  RoadInfoBusReader/4 -> Subsystem/2(In2)  "Y"
  RoadInfoBusReader/5 -> Subsystem/3(In3)  "Z"
  RoadInfoBusReader/6 -> Subsystem/4(In4)  "dzdx"
  RoadInfoBusReader/7 -> Subsystem/5(In6)  "dzdy"
  RoadInfoBusReader/8 -> Subsystem/6(In5)  "mu"
  Subsystem/4(mu) -> MATLAB Function1/5(mu)
  Subsystem/3(dzdy) -> MATLAB Function1/4(dzdy)
  Subsystem/1(z) -> MATLAB Function1/2(z)
  Subsystem/2(dzdx) -> MATLAB Function1/3(dzdx)
  MATLAB Function/2(tire_y) -> Subsystem1/2(Ry_eo2ctc_coE_Refine), TireY/1  "Ry_eo2ctc_coE_Refine"
  MATLAB Function/1(tire_x) -> Subsystem1/1(Rx_eo2ctc_coE_Refine), TireX/1  "Rx_eo2ctc_coE_Refine"
  Subsystem1/1(P1) -> Subsystem/7(P1)
  Subsystem1/2(P2) -> Subsystem/8(P2)
  Subsystem1/3(P3) -> Subsystem/9(P3)
  Subsystem1/4(P4) -> Subsystem/10(P4)

== system LKASampleSimulink/Veh_1/DriverModel/DriverFilter ==
  note: DriverBusCreator
  Bus Creator2 : BusCreator  Inputs=6
  Bus Selector : BusSelector  OutputSignals=valid,throttle,brake,steer,mode,gear
  Data Store Write : DataStoreWrite  DataStoreName=DataStore_Ego_Control
  EgoControlBus : S-Function  FunctionName=BusReader  Parameters='ego_control','time@i,valid@b,throttle@d,brake@d,steer@d,mode@i,gear@i','0.001','0.0'  SFunctionDeploymentMode=off  EnableBusSupport=off
  Gain : Gain  OutDataTypeStr=double
  Gain1 : Gain  OutDataTypeStr=double
  Gain2 : Gain  OutDataTypeStr=double
  Mux : Mux  Inputs=6
  DriverOut : Outport  VectorParamsAs1DForOutWhenUnconnected=off
  wires:
  Bus Selector/6 -> Gain1/1  "<gear>"
  Bus Selector/1 -> Gain2/1  "<valid>"
  Bus Creator2/1 -> DriverOut/1, Bus Selector/1
  Gain/1 -> Mux/5
  Bus Selector/2 -> Mux/2  "<throttle>"
  Bus Selector/5 -> Gain/1  "<mode>"
  Gain1/1 -> Mux/6
  Gain2/1 -> Mux/1
  Bus Selector/4 -> Mux/4  "<steer>"
  Mux/1 -> Data Store Write/1
  Bus Selector/3 -> Mux/3  "<brake>"
  EgoControlBus/4 -> Bus Creator2/3  "brake"
  EgoControlBus/5 -> Bus Creator2/4  "steer"
  EgoControlBus/3 -> Bus Creator2/2  "throttle"
  EgoControlBus/2 -> Bus Creator2/1  "valid"
  EgoControlBus/6 -> Bus Creator2/5  "mode"
  EgoControlBus/7 -> Bus Creator2/6  "gear"

== system LKASampleSimulink/Veh_1/GlobalVariable/Variable ==
  GlobalVariable0 : S-Function  FunctionName=BusReader  Parameters='global.0','time@i,variable@d','0.01','0.0'  SFunctionDeploymentMode=off  EnableBusSupport=off
  GlobalVariable1 : S-Function  FunctionName=BusReader  Parameters='global.1','time@i,variable@d','0.01','0.0'  SFunctionDeploymentMode=off  EnableBusSupport=off
  GlobalVariable2 : S-Function  FunctionName=BusReader  Parameters='global.2','time@i,variable@d','0.01','0.0'  SFunctionDeploymentMode=off  EnableBusSupport=off
  GlobalVariable3 : S-Function  FunctionName=BusReader  Parameters='global.3','time@i,variable@d','0.01','0.0'  SFunctionDeploymentMode=off  EnableBusSupport=off
  GlobalVariable4 : S-Function  FunctionName=BusReader  Parameters='global.4','time@i,variable@d','0.01','0.0'  SFunctionDeploymentMode=off  EnableBusSupport=off
  GlobalVariable5 : S-Function  FunctionName=BusReader  Parameters='global.5','time@i,variable@d','0.01','0.0'  SFunctionDeploymentMode=off  EnableBusSupport=off
  GlobalVariable6 : S-Function  FunctionName=BusReader  Parameters='global.6','time@i,variable@d','0.01','0.0'  SFunctionDeploymentMode=off  EnableBusSupport=off
  GlobalVariable7 : S-Function  FunctionName=BusReader  Parameters='global.7','time@i,variable@d','0.01','0.0'  SFunctionDeploymentMode=off  EnableBusSupport=off
  GlobalVariable8 : S-Function  FunctionName=BusReader  Parameters='global.8','time@i,variable@d','0.01','0.0'  SFunctionDeploymentMode=off  EnableBusSupport=off
  GlobalVariable9 : S-Function  FunctionName=BusReader  Parameters='global.9','time@i,variable@d','0.01','0.0'  SFunctionDeploymentMode=off  EnableBusSupport=off
  Mux : Mux  Inputs=10
  Mux1 : Mux  Inputs=10
  Out1 : Outport  VectorParamsAs1DForOutWhenUnconnected=off
  Out2 : Outport  Port=2  VectorParamsAs1DForOutWhenUnconnected=off
  wires:
  GlobalVariable9/1 -> Mux1/10
  GlobalVariable8/1 -> Mux1/9
  GlobalVariable7/1 -> Mux1/8
  GlobalVariable6/1 -> Mux1/7
  GlobalVariable5/1 -> Mux1/6
  GlobalVariable4/1 -> Mux1/5
  GlobalVariable3/1 -> Mux1/4
  GlobalVariable2/1 -> Mux1/3
  GlobalVariable1/1 -> Mux1/2
  GlobalVariable0/1 -> Mux1/1
  Mux1/1 -> Out2/1
  GlobalVariable9/2 -> Mux/10
  GlobalVariable8/2 -> Mux/9
  GlobalVariable7/2 -> Mux/8
  GlobalVariable6/2 -> Mux/7
  GlobalVariable5/2 -> Mux/6
  GlobalVariable4/2 -> Mux/5
  GlobalVariable3/2 -> Mux/4
  GlobalVariable2/2 -> Mux/3
  GlobalVariable1/2 -> Mux/2
  Mux/1 -> Out1/1
  GlobalVariable0/2 -> Mux/1

== system LKASampleSimulink/Veh_1/Sensors/GroundTruth_Objects.0 ==
  BusCreator : BusCreator  Inputs=time,width,id,type,shape,range_center,range_bbox,azimuth_angle,elevation_angle,velocity,heading
  SensorBus : S-Function  FunctionName=BusReader  Parameters='GroundTruth_Objects.0','time@i,100@[,id@i,type@b,shape@i,range_center@f,range_bbox@f,azimuth_angle@f,elevation_angle@f,velocity@f,heading@f','0.01','0.0'  SFunctionDeploymentMode=off  EnableBusSupport=off
  SensorOut : Outport  VectorParamsAs1DForOutWhenUnconnected=off
  wires:
  SensorBus/11 -> BusCreator/11  "heading"
  SensorBus/10 -> BusCreator/10  "velocity"
  SensorBus/9 -> BusCreator/9  "elevation_angle"
  SensorBus/8 -> BusCreator/8  "azimuth_angle"
  SensorBus/7 -> BusCreator/7  "range_bbox"
  SensorBus/6 -> BusCreator/6  "range_center"
  SensorBus/5 -> BusCreator/5  "shape"
  SensorBus/4 -> BusCreator/4  "type"
  SensorBus/3 -> BusCreator/3  "id"
  SensorBus/2 -> BusCreator/2  "width"
  SensorBus/1 -> BusCreator/1  "time"
  BusCreator/1 -> SensorOut/1

== system LKASampleSimulink/Veh_1/Sensors/LaneInfoPerception.0 ==
  BusCreator : BusCreator  Inputs=Timestamp,width,Lane_ID,Lane_Distance,Lane_Car_Distance_Left,Lane_Car_Distance_Right,Lane_Curvature,Lane_Coefficient_C0,Lane_Coefficient_C1,Lane_Coefficient_C2,Lane_Coefficient_C3,Lane_Class
  SensorBus : S-Function  FunctionName=BusReader  Parameters='LaneInfoPerception.0','Timestamp@i,4@[,Lane_ID@i,Lane_Distance@d,Lane_Car_Distance_Left@d,Lane_Car_Distance_Right@d,Lane_Curvature@d,Lane_Coefficient_C0@d,Lane_Coefficient_C1@d,Lane_Coefficient_C2@d,Lane_Coefficient_C3@d,Lane_Class@b','0.01','0.0'  SFunctionDeploymentMode=off  EnableBusSupport=off
  SensorOut : Outport  VectorParamsAs1DForOutWhenUnconnected=off
  wires:
  SensorBus/12 -> BusCreator/12  "Lane_Class"
  SensorBus/11 -> BusCreator/11  "Lane_Coefficient_C3"
  SensorBus/10 -> BusCreator/10  "Lane_Coefficient_C2"
  SensorBus/9 -> BusCreator/9  "Lane_Coefficient_C1"
  SensorBus/8 -> BusCreator/8  "Lane_Coefficient_C0"
  SensorBus/7 -> BusCreator/7  "Lane_Curvature"
  SensorBus/6 -> BusCreator/6  "Lane_Car_Distance_Right"
  SensorBus/5 -> BusCreator/5  "Lane_Car_Distance_Left"
  SensorBus/4 -> BusCreator/4  "Lane_Distance"
  SensorBus/3 -> BusCreator/3  "Lane_ID"
  SensorBus/2 -> BusCreator/2  "width"
  SensorBus/1 -> BusCreator/1  "Timestamp"
  BusCreator/1 -> SensorOut/1

== system LKASampleSimulink/Veh_1/Sensors/sensor_template ==
  BusCreator : BusCreator  Inputs=8
  SensorBus : S-Function  FunctionName=BusReader  Parameters='mmwradar.0','time@i,64@[,angle@d,distance@d,speed@d,type@b,energy@d,id@i','0.1','0.0'  SFunctionDeploymentMode=off  EnableBusSupport=off
  SensorOut : Outport  VectorParamsAs1DForOutWhenUnconnected=off
  wires:
  BusCreator/1 -> SensorOut/1

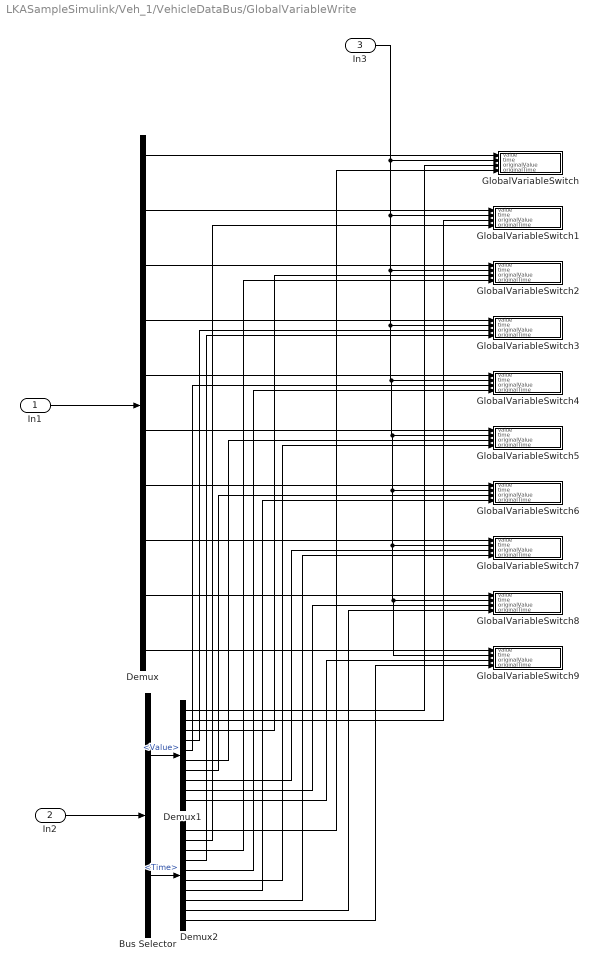
== system LKASampleSimulink/Veh_1/VehicleDataBus/GlobalVariableWrite ==
  In1 : Inport
  In2 : Inport  Port=2
  In3 : Inport  Port=3
  Bus Selector : BusSelector  OutputSignals=Value,Time
  Demux : Demux  Outputs=10
  Demux1 : Demux  Outputs=10
  Demux2 : Demux  Outputs=10
  GlobalVariableSwitch : Subsystem
  GlobalVariableSwitch1 : Subsystem
  GlobalVariableSwitch2 : Subsystem
  GlobalVariableSwitch3 : Subsystem
  GlobalVariableSwitch4 : Subsystem
  GlobalVariableSwitch5 : Subsystem
  GlobalVariableSwitch6 : Subsystem
  GlobalVariableSwitch7 : Subsystem
  GlobalVariableSwitch8 : Subsystem
  GlobalVariableSwitch9 : Subsystem
  wires:
  Demux2/10 -> GlobalVariableSwitch9/4(originalTime)
  Demux1/10 -> GlobalVariableSwitch9/3(originalValue)
  Demux/10 -> GlobalVariableSwitch9/1(value)
  Demux2/9 -> GlobalVariableSwitch8/4(originalTime)
  Demux1/9 -> GlobalVariableSwitch8/3(originalValue)
  Demux/9 -> GlobalVariableSwitch8/1(value)
  Demux2/8 -> GlobalVariableSwitch7/4(originalTime)
  Demux1/8 -> GlobalVariableSwitch7/3(originalValue)
  Demux/8 -> GlobalVariableSwitch7/1(value)
  Demux2/7 -> GlobalVariableSwitch6/4(originalTime)
  Demux1/7 -> GlobalVariableSwitch6/3(originalValue)
  Demux/7 -> GlobalVariableSwitch6/1(value)
  Demux2/6 -> GlobalVariableSwitch5/4(originalTime)
  Demux1/6 -> GlobalVariableSwitch5/3(originalValue)
  Demux/6 -> GlobalVariableSwitch5/1(value)
  Demux2/5 -> GlobalVariableSwitch4/4(originalTime)
  Demux1/5 -> GlobalVariableSwitch4/3(originalValue)
  Demux/5 -> GlobalVariableSwitch4/1(value)
  Demux2/4 -> GlobalVariableSwitch3/4(originalTime)
  Demux1/4 -> GlobalVariableSwitch3/3(originalValue)
  Demux/4 -> GlobalVariableSwitch3/1(value)
  Demux2/3 -> GlobalVariableSwitch2/4(originalTime)
  Demux1/3 -> GlobalVariableSwitch2/3(originalValue)
  Demux/3 -> GlobalVariableSwitch2/1(value)
  Demux2/2 -> GlobalVariableSwitch1/4(originalTime)
  Demux1/2 -> GlobalVariableSwitch1/3(originalValue)
  Demux/2 -> GlobalVariableSwitch1/1(value)
  Demux2/1 -> GlobalVariableSwitch/4(originalTime)
  Demux1/1 -> GlobalVariableSwitch/3(originalValue)
  Demux/1 -> GlobalVariableSwitch/1(value)
  Bus Selector/2 -> Demux2/1  "<Time>"
  Bus Selector/1 -> Demux1/1  "<Value>"
  In2/1 -> Bus Selector/1
  In1/1 -> Demux/1
  In3/1 -> GlobalVariableSwitch/2(time), GlobalVariableSwitch1/2(time), GlobalVariableSwitch2/2(time), GlobalVariableSwitch3/2(time), GlobalVariableSwitch4/2(time), GlobalVariableSwitch5/2(time), GlobalVariableSwitch6/2(time), GlobalVariableSwitch7/2(time), GlobalVariableSwitch8/2(time), GlobalVariableSwitch9/2(time)

== system LKASampleSimulink/Veh_1/Algorithm/lane Following Controller/Controller Mode Selector ==
  note: Input: Deceleration, Watchdog Brake, Acceleration
      | Description: based on the watchdog brake, either select acceleration computed from the controller or the deceleration from the watchdog controller
      | Output: Acceleration Cmd
  Acceleration : Inport
  WatchdogBrake : Inport  Port=2
  Deceleration : Inport  Port=3
  Constant1 : Constant  Value=BrStatus.NoBrake  OutDataTypeStr=Enum: BrStatus
  GreaterThan1 : RelationalOperator  Operator=>  RndMeth=Simplest
  Saturation : Saturate  UpperLimit=2  LowerLimit=-10
      settings: AttributesFormatString=|
      | %<UpperLimit>
      | %<LowerLimit>
  Switch : Switch  Criteria=u2 ~= 0
  UnaryMinus : UnaryMinus
  AccelerationCmd : Outport
  wires:
  Switch/1 -> Saturation/1
  WatchdogBrake/1 -> GreaterThan1/1  "braking_switch"
  UnaryMinus/1 -> Switch/1
  Deceleration/1 -> UnaryMinus/1  "wdg_deceleration"
  Saturation/1 -> AccelerationCmd/1
  Acceleration/1 -> Switch/3  "mpc_acceleration"
  Constant1/1 -> GreaterThan1/2
  GreaterThan1/1 -> Switch/2

== system LKASampleSimulink/Veh_1/Algorithm/lane Following Controller/MPC Controller ==
  note: Input: SetVelocity, LongitudinalVelocity, Curvature, LateralDeviation, RelativeYawAngle, RelativeDistanc, RelativeVelocity
      | Description: based on inputs, decide on optimal Accerlation and SteeringAngle to output
      | Output: SteeringAngle, Acceleration
  Set velocity : Inport
  Longitudinal velocity : Inport  Port=2
  Curvature : Inport  Port=3
  Lateral deviation : Inport  Port=4
  Relative yaw angle : Inport  Port=5
  Relative distance : Inport  Port=6
  Relative velocity : Inport  Port=7
  InValueLimiters : Subsystem
  Path Following Control System : mpcadaslib/Path Following Control System  VariantControl=Variant2  ModelType=Use vehicle parameters  VehicleMass=1575  VehicleYawInertia=2875  LengthToFront=1.5130000000000001  LengthToRear=1.305  FrontTireStiffness=19000  RearTireStiffness=33000  AccelTimeConstant=0.5  EgoModelMatrixA=[-2,zeros(1,3);1,zeros(1,3);zeros(1,2),-4.4021,-12.4603;zeros(1,2),1.3913,-5.1868]  EgoModelMatrixB=[2,zeros(1,3);zeros(1,2),24.1270,15.8609]'  EgoModelMatrixC=[zeros(3,1),eye(3)]  InitialLongVel=14.0  TransportLag=0.1  spaceCtrl=on  DefaultSpacing=10  MinSteering=-0.26  umin_ext=off  MaxSteering=0.26  umax_ext=off  MinAcceleration=-3  amin_ext=off  MaxAcceleration=2  amax_ext=off  Ts=0.1  PredictionHorizon=30  ControlHorizon=2  LongWeight=0.1  LateralWeight=1  AccelRateWeight=0.1  SteerRateWeight=0.1  suboptimal=off  maxiter=10  datatypeopt=double  optmode=off  trackmode=off
      settings: SourceProductBaseCode=MP
  time_gap : Constant  Value=1.5
  Steering Angle : Outport  VectorParamsAs1DForOutWhenUnconnected=off
  Acceleration : Outport  Port=2  VectorParamsAs1DForOutWhenUnconnected=off
  wires:
  time_gap/1 -> Path Following Control System/2
  Relative yaw angle/1 -> Path Following Control System/8
  Lateral deviation/1 -> Path Following Control System/7
  Curvature/1 -> Path Following Control System/6
  Set velocity/1 -> Path Following Control System/1
  Path Following Control System/2 -> Steering Angle/1
  Path Following Control System/1 -> Acceleration/1
  Longitudinal velocity/1 -> InValueLimiters/3(LongitudinalVelocityIn)
  Relative distance/1 -> InValueLimiters/1(RelativeDistanceIn)
  Relative velocity/1 -> InValueLimiters/2(RelativeVelocityIn)
  InValueLimiters/1(Relative distance) -> Path Following Control System/3
  InValueLimiters/2(Relative velocity) -> Path Following Control System/4
  InValueLimiters/3(Longitudinal velocity) -> Path Following Control System/5

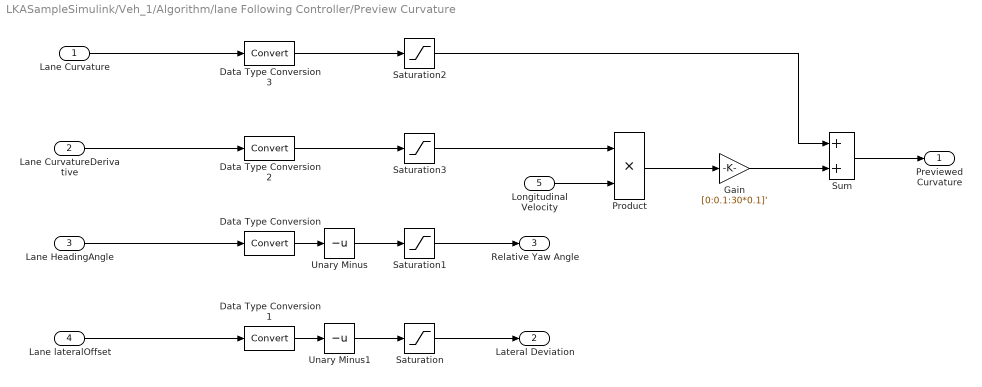
== system LKASampleSimulink/Veh_1/Algorithm/lane Following Controller/Preview Curvature ==
  Lane Curvature : Inport
  Lane CurvatureDerivative : Inport  Port=2
  Lane HeadingAngle : Inport  Port=3
  Lane lateralOffset : Inport  Port=4
  Longitudinal Velocity : Inport  Port=5
  Data Type Conversion{,1..3} (4 alike) : DataTypeConversion
  Gain : Gain  Gain=[0:0.1:30*0.1]'
      settings: AttributesFormatString=|
      | ----------------------------------------
      | Gain = %<Gain>
  Product : Product
  Saturation : Saturate
      settings: AttributesFormatString=|
      | -------------------------------
      | UpperLimit = %<UpperLimit>
      | LowerLimit = %<LowerLimit>
  Saturation1 : Saturate  UpperLimit=0.6  LowerLimit=-0.6
      settings: AttributesFormatString=|
      | -------------------------------
      | UpperLimit = %<UpperLimit>
      | LowerLimit = %<LowerLimit>
  Saturation2 : Saturate  UpperLimit=0.15  LowerLimit=-0.15
      settings: AttributesFormatString=|
      | -------------------------------
      | UpperLimit = %<UpperLimit>
      | LowerLimit = %<LowerLimit>
  Saturation3 : Saturate  UpperLimit=0.06  LowerLimit=-0.06
      settings: AttributesFormatString=|
      | -------------------------------
      | UpperLimit = %<UpperLimit>
      | LowerLimit = %<LowerLimit>
  Sum : Sum
  Unary Minus : UnaryMinus
  Unary Minus1 : UnaryMinus
  Previewed Curvature : Outport  VectorParamsAs1DForOutWhenUnconnected=off
  Lateral Deviation : Outport  Port=2  VectorParamsAs1DForOutWhenUnconnected=off
  Relative Yaw Angle : Outport  Port=3  VectorParamsAs1DForOutWhenUnconnected=off
  wires:
  Lane HeadingAngle/1 -> Data Type Conversion/1
  Lane lateralOffset/1 -> Data Type Conversion1/1
  Unary Minus1/1 -> Saturation/1
  Lane Curvature/1 -> Data Type Conversion3/1
  Lane CurvatureDerivative/1 -> Data Type Conversion2/1
  Longitudinal Velocity/1 -> Product/2
  Unary Minus/1 -> Saturation1/1
  Saturation/1 -> Lateral Deviation/1
  Saturation1/1 -> Relative Yaw Angle/1
  Saturation3/1 -> Product/1
  Product/1 -> Gain/1
  Sum/1 -> Previewed Curvature/1
  Gain/1 -> Sum/2
  Saturation2/1 -> Sum/1
  Data Type Conversion/1 -> Unary Minus/1
  Data Type Conversion1/1 -> Unary Minus1/1
  Data Type Conversion2/1 -> Saturation3/1
  Data Type Conversion3/1 -> Saturation2/1

== system LKASampleSimulink/Veh_1/Algorithm/lane Following Controller/Watchdog Braking Controller ==
  Longitudinal Velocity : Inport
  MIO Relative Distance : Inport  Port=2
  MIO Relative Velocity : Inport  Port=3
  BrakeTimeCalculation : Subsystem
  BrakingLogic : Subsystem
  FB_decel : Constant  Value=9.8
  PB1_decel : Constant  Value=3.8
  PB2_decel : Constant  Value=5.3
  TTCCalculation : Subsystem
  Brake Status : Outport  VectorParamsAs1DForOutWhenUnconnected=off
  Deceleration : Outport  Port=2  VectorParamsAs1DForOutWhenUnconnected=off
  wires:
  BrakingLogic/2(decel) -> Deceleration/1
  BrakingLogic/1(BrakeStatus) -> Brake Status/1
  MIO Relative Distance/1 -> BrakingLogic/1(relativeDistance), TTCCalculation/1(mioDistance)
  MIO Relative Velocity/1 -> TTCCalculation/2(mioVelocity)
  TTCCalculation/1(TTC) -> BrakingLogic/2(TTC)
  Longitudinal Velocity/1 -> BrakingLogic/7(longVelocity), BrakeTimeCalculation/4(LongitudinalVelocity)
  PB1_decel/1 -> BrakeTimeCalculation/1(PB1Decel)
  PB2_decel/1 -> BrakeTimeCalculation/2(PB2Decel)
  FB_decel/1 -> BrakeTimeCalculation/3(FBDecel)
  BrakeTimeCalculation/1(FCWstoppingTime) -> BrakingLogic/3(FCWtime)
  BrakeTimeCalculation/2(PB1stoppingTime) -> BrakingLogic/4(PB1time)
  BrakeTimeCalculation/3(PB2stoppingTime) -> BrakingLogic/5(PB2time)
  BrakeTimeCalculation/4(FBstoppingTime) -> BrakingLogic/6(FBtime)
